simulink model "Taller1_SCADA"  (R2024a)
settings: Solver=VariableStepAuto  StartTime=0.0  StopTime=inf  RelTol=1e-3
libraries: spsThreePhaseTransformerTwoWindingsLib x2, spsThreePhaseVIMeasurementLib x2, spsPower3phInstantaneousLib x2, spsAsynchronousMachinepuUnitsLib x1, spsThreePhaseParallelRLCLoadLib x1, spsThreePhaseSeriesRLCBranchLib x1, spsThreePhaseBreakerLib x1, spsThreePhaseSourceLib x1, spsRMSLib x1, spspowerguiLib x1
settings Model: Creator=estudiante  LastModifiedBy=danan
settings SolverCC: AlgebraicLoopSolver=TrustRegion
settings DataIOCC: ReturnWorkspaceOutputs=off
settings DebuggingCC: UnconnectedInputMsg=warning  UnconnectedOutputMsg=warning  UnconnectedLineMsg=warning  ArithmeticOperatorsInVariantConditions=warning
settings ModelReferenceCC: EnableRefExpFcnMdlSchedulingChecks=on
settings SFSimCC: SimUseLocalCustomCode=off  CustomCodeUndefinedFunction=UseInterfaceOnly
settings RTWCC: RTWUseLocalCustomCode=off  GPUComputeCapability=3.5
settings CodeAppCC: StateflowObjectComments=on
settings SimscapeCC: SimscapeNormalizeSystem=off

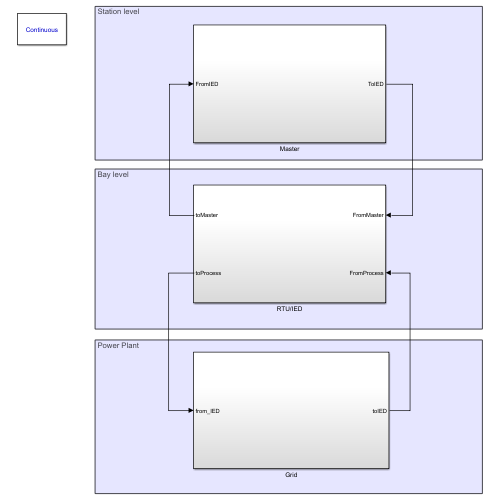
[thumbnail: Simulink's stored preview of the top-level diagram]
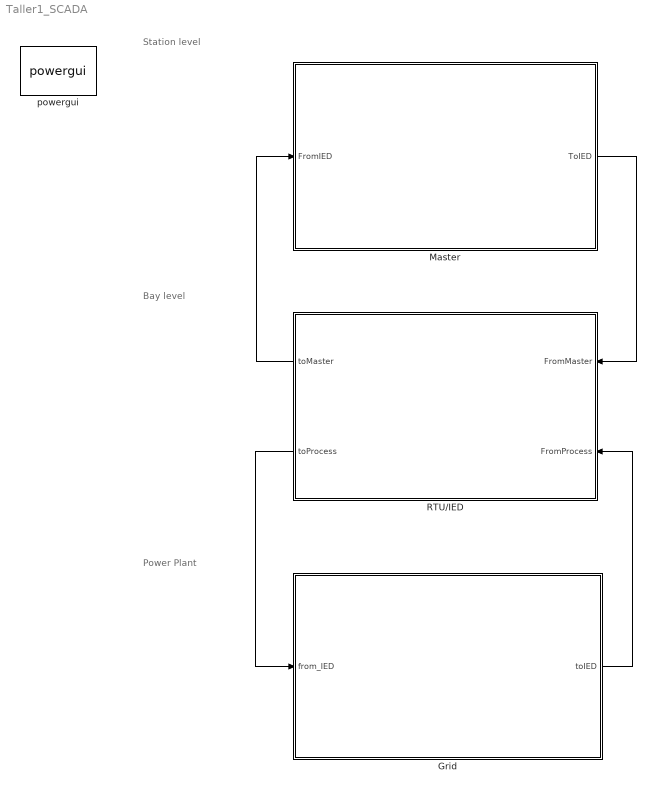
== system Taller1_SCADA ==
  note: Station level
  note: Bay level
  note: Power Plant
  Grid : Subsystem
  Master : Subsystem
  RTU/IED : Subsystem
  powergui : spspowerguiLib/powergui  Priority=1  SimulationMode=Continuous  SampleTime=50e-6  frequency=60  Iterations=50  frequencyindice=60  Pbase=100e6  ErrMax=1e-4  UnitsV=kV  UnitsW=MW  buscounter=0  FunctionMessages=off  echomessages=off  EnableUseOfTLC=off  CurrentSourceSwitches=off  DisableSnubberDevices=off  DisableRonSwitches=off  DisableVfSwitches=off  DisplayEquations=off  AutomaticDiscreteSolvers=off  SolverType=Tustin/Backward Euler (TBE)  Interpol=off  ExternalGateDelay=off  methode=off  Ts=10  x0status=blocks  SPID=off  SwTol=0  HookPort=off  NonlinearTolerance=1e-4  nMaxIteration=100  ContinueOnMaxIteration=off  RestoreLinks=warning  ResistiveCurrentMeasurement=off  Frange=[0:2:500]  Ylog=off  Xlog=on  ShowGrid=off  save=off  variable=ZData  structure=0  ZoomFFT=off  StartTime=0.0  cycles=1  DisplayStyle=1  fundamental=60  FreqAxis=off  MaxFrequency=1000  frequencyindicesteady=1  RmsSteady=1  display=off
  wires:
  RTU/IED/2(toProcess) -> Grid/1(from_IED)
  Grid/1(toIED) -> RTU/IED/2(FromProcess)
  RTU/IED/1(toMaster) -> Master/1(FromIED)
  Master/1(ToIED) -> RTU/IED/1(FromMaster)

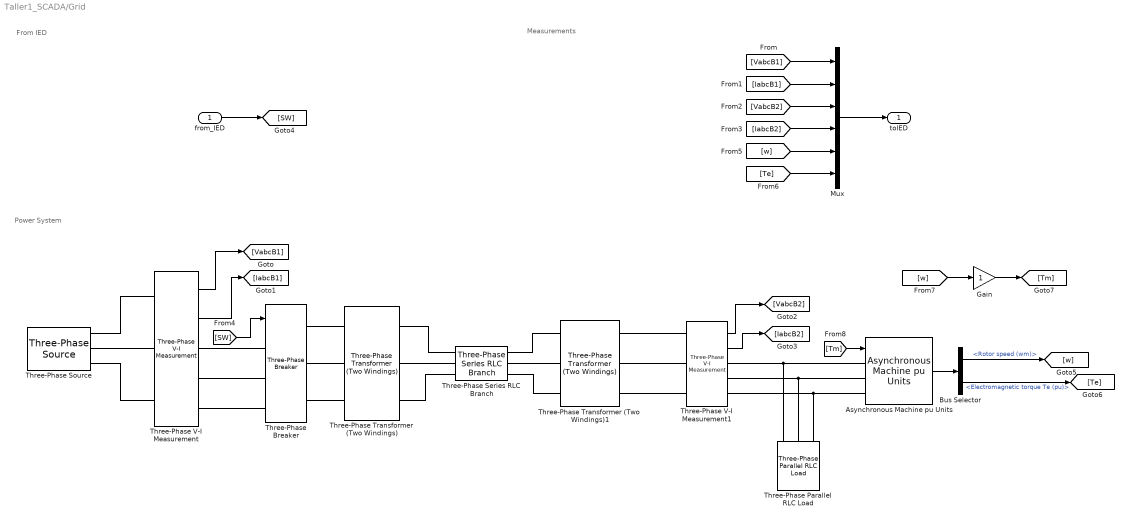
== system Taller1_SCADA/Grid ==
  note: From IED
  note: Measurements
  note: Power System
  from_IED : Inport
  Asynchronous Machine pu Units : spsAsynchronousMachinepuUnitsLib/Asynchronous Machine pu Units  RotorType=Squirrel-cage  PresetModel=No  MechanicalLoad=Torque Tm  ShowDetailedParameters=on  ReferenceFrame=Rotor  Units=pu  MeasurementBus=off  NominalParameters=[3730 460 60]  VoltageRatio=1  Stator=[0.01965 0.0397]  Rotor=[0.01909 0.0397]  Cage1=[0.01909 0.0397]  Cage2=[0.01909 0.0397]  Lm=1.354  Mechanical=[0.09526 0.05479 2]  PolePairs=2  InitialConditions="[ 1,0   0,0,0   0,0,0 ]"  SimulateSaturation=off  Saturation="[0.212,0.4201,0.8125,1.0979,1.4799,2.2457,3.2586,4.5763,6.4763 ;   0.5,0.7,0.9,1,1.1,1.2 ,1.3,1.4,1.5]"  LoadFlowParameters=0  TsPowergui=0  TsBlock=-1  IterativeModel=Trapezoidal non iterative  IterativeDiscreteModel=Trapezoidal non iterative  Pmec=0
      settings: LibrarySourceBlock=|
      | sps_lib/Electrical Machines/Asynchronous Machine
      | pu Units
  Bus Selector : BusSelector  OutputSignals=Mechanical.Rotor speed (wm),Mechanical.Electromagnetic torque Te (pu)
  Gain : Gain
  Mux : Mux  Inputs=6
  Three-Phase Parallel RLC Load : spsThreePhaseParallelRLCLoadLib/Three-Phase Parallel RLC Load  LConnTagsString=A|B|C  Configuration=Y (grounded)  NominalVoltage=1000  Vabc=[1e3 1e3 1e3]  Vabcp=[1e3 1e3 1e3]  NominalFrequency=60  UnbalancedPower=off  ActivePower=10e3  InductivePower=100  CapacitivePower=100  Pabc=[10e3 9e3 11e3]  QLabc=[100 90 110]  QCabc=[100 90 110]  Pabcp=[10e3 9e3 11e3]  QLabcp=[100 90 110]  QCabcp=[100 90 110]  Measurements=None  LoadType=constant Z
  Three-Phase Series RLC Branch : spsThreePhaseSeriesRLCBranchLib/Three-Phase Series RLC Branch  LConnTagsString=A|B|C  RConnTagsString=A|B|C  BranchType=RLC  Resistance=1  Inductance=1e-3  Capacitance=1e-6  Measurements=None
  Three-Phase Transformer (Two Windings) : spsThreePhaseTransformerTwoWindingsLib/Three-Phase Transformer (Two Windings)  Winding1Connection=Yg  Winding2Connection=Yg  CoreType=Three single-phase transformers  SetSaturation=off  Hysteresis=off  DataFile='hysteresis'  SetInitialFlux=off  Measurements=None  UNITS=pu  NominalPower=[ 250e6 , 60 ]  Winding1=[ 735e3 , 0.002 , 0.08 ]  Winding2=[ 315e3 , 0.002 , 0.08 ]  Rm=500  Lm=500  L0=0.5  Saturation=[ 0,0 ; 0.0024,1.2 ; 1.0,1.52 ]  InitialFluxes=[ 0.8 , -0.8 , 0.7 ]  BreakLoop=off  DiscreteSolver=Trapezoidal iterative  DataType=off  TransfoNumber=1
  Three-Phase Transformer (Two Windings)1 : spsThreePhaseTransformerTwoWindingsLib/Three-Phase Transformer (Two Windings)  Winding1Connection=Yg  Winding2Connection=Yg  CoreType=Three single-phase transformers  SetSaturation=off  Hysteresis=off  DataFile='hysteresis'  SetInitialFlux=off  Measurements=None  UNITS=pu  NominalPower=[ 250e6 , 60 ]  Winding1=[ 735e3 , 0.002 , 0.08 ]  Winding2=[ 315e3 , 0.002 , 0.08 ]  Rm=500  Lm=500  L0=0.5  Saturation=[ 0,0 ; 0.0024,1.2 ; 1.0,1.52 ]  InitialFluxes=[ 0.8 , -0.8 , 0.7 ]  BreakLoop=off  DiscreteSolver=Trapezoidal iterative  DataType=off  TransfoNumber=1
  Three-Phase V-I Measurement : spsThreePhaseVIMeasurementLib/Three-Phase V-I Measurement  VoltageMeasurement=phase-to-ground  SetLabelV=off  LabelV=Vabc  Vpu=off  VpuLL=off  CurrentMeasurement=yes  SetLabelI=off  LabelI=Iabc  Ipu=off  Pbase=100e6  Vbase=500e3  OutputType=Complex  PhasorSimulation=off  PSBequivalent=0
  Three-Phase V-I Measurement1 : spsThreePhaseVIMeasurementLib/Three-Phase V-I Measurement  VoltageMeasurement=phase-to-ground  SetLabelV=off  LabelV=Vabc  Vpu=off  VpuLL=off  CurrentMeasurement=yes  SetLabelI=off  LabelI=Iabc  Ipu=off  Pbase=100e6  Vbase=500e3  OutputType=Complex  PhasorSimulation=off  PSBequivalent=0
  Three-Phase Breaker : spsThreePhaseBreakerLib/Three-Phase Breaker  InitialState=open  SwitchA=on  SwitchB=on  SwitchC=on  SwitchTimes="[1/60  5/60]"  External=on  BreakerResistance=0.01  SnubberResistance=1e6  SnubberCapacitance=inf  Measurements=None
  Three-Phase Source : spsThreePhaseSourceLib/Three-Phase Source  InternalConnection=Yg  VoltagePhases=off  Voltage=25e3  PhaseAngle=0  Voltage_phases=[25e3 25e3 25e3]/sqrt(3)  PhaseAngles_phases=[0 -120 +120]  Frequency=60  NonIdealSource=on  SpecifyImpedance=off  Resistance=0.8929  Inductance=16.58e-3  ShortCircuitLevel=100e6  BaseVoltage=25e3  XRratio=7  BusType=swing  Pref=10e3  Qref=0  Prefabc=[10e3, 10e3, 10e3]  Qrefabc=[0, 0, 0]  Qmin=-inf  Qmax=inf
  toIED : Outport
  wires:
  Three-Phase V-I Measurement/1 -> [VabcB1]
  Three-Phase V-I Measurement/2 -> [IabcB1]
  Three-Phase V-I Measurement1/2 -> [IabcB2]
  Three-Phase V-I Measurement1/1 -> [VabcB2]
  Asynchronous Machine pu Units/1 -> Bus Selector/1
  [SW] -> Three-Phase Breaker/1
  Bus Selector/1 -> [w]  "<Rotor speed (wm)>"
  Bus Selector/2 -> [Te]  "<Electromagnetic torque Te (pu)>"
  from_IED/1 -> [SW]
  Mux/1 -> toIED/1
  [VabcB1] -> Mux/1
  [IabcB1] -> Mux/2
  [VabcB2] -> Mux/3
  [IabcB2] -> Mux/4
  [w] -> Mux/5
  [Te] -> Mux/6
  [w] -> Gain/1
  Gain/1 -> [Tm]
  [Tm] -> Asynchronous Machine pu Units/1
  connections:
  Three-Phase V-I Measurement/RConn3 -- Three-Phase Breaker/LConn3
  Three-Phase Transformer (Two Windings)/LConn1 -- Three-Phase Breaker/RConn1
  Three-Phase Source/RConn2 -- Three-Phase V-I Measurement/LConn2
  Three-Phase Breaker/RConn3 -- Three-Phase Transformer (Two Windings)/LConn3
  Three-Phase Transformer (Two Windings)/LConn2 -- Three-Phase Breaker/RConn2
  Three-Phase Transformer (Two Windings)1/LConn2 -- Three-Phase Series RLC Branch/RConn2
  Three-Phase Series RLC Branch/LConn1 -- Three-Phase Transformer (Two Windings)/RConn1
  Three-Phase Source/RConn1 -- Three-Phase V-I Measurement/LConn1
  Three-Phase Series RLC Branch/RConn1 -- Three-Phase Transformer (Two Windings)1/LConn1
  Three-Phase Source/RConn3 -- Three-Phase V-I Measurement/LConn3
  Three-Phase V-I Measurement/RConn1 -- Three-Phase Breaker/LConn1
  Three-Phase V-I Measurement/RConn2 -- Three-Phase Breaker/LConn2
  Three-Phase Series RLC Branch/LConn2 -- Three-Phase Transformer (Two Windings)/RConn2
  Three-Phase Series RLC Branch/LConn3 -- Three-Phase Transformer (Two Windings)/RConn3
  Three-Phase Series RLC Branch/RConn3 -- Three-Phase Transformer (Two Windings)1/LConn3
  Asynchronous Machine pu Units/LConn1 -- Three-Phase Parallel RLC Load/LConn1 -- Three-Phase V-I Measurement1/RConn1
  Asynchronous Machine pu Units/LConn2 -- Three-Phase Parallel RLC Load/LConn2 -- Three-Phase V-I Measurement1/RConn2
  Asynchronous Machine pu Units/LConn3 -- Three-Phase Parallel RLC Load/LConn3 -- Three-Phase V-I Measurement1/RConn3
  Three-Phase V-I Measurement1/LConn1 -- Three-Phase Transformer (Two Windings)1/RConn1
  Three-Phase V-I Measurement1/LConn2 -- Three-Phase Transformer (Two Windings)1/RConn2
  Three-Phase V-I Measurement1/LConn3 -- Three-Phase Transformer (Two Windings)1/RConn3

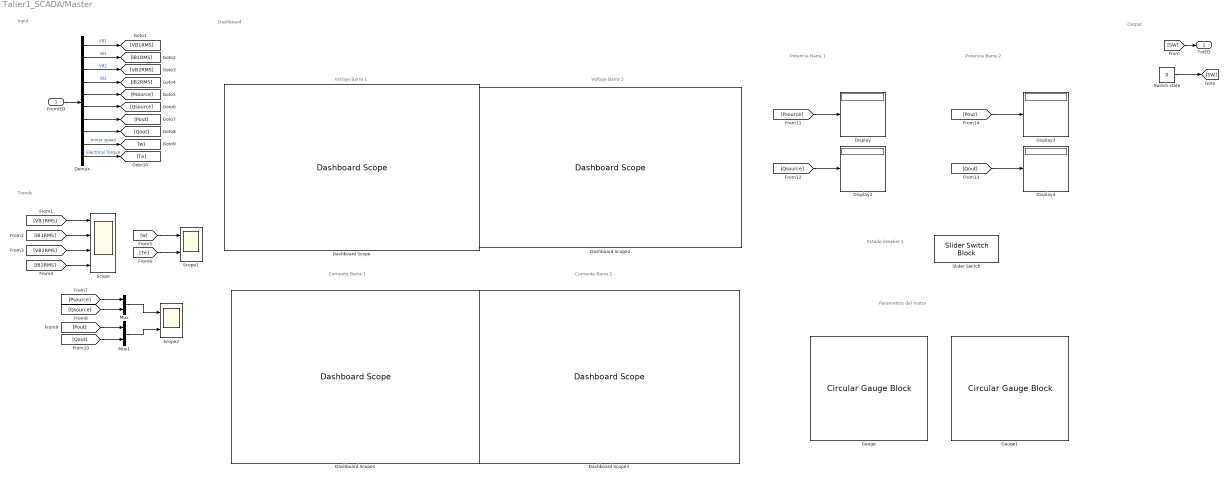
== system Taller1_SCADA/Master ==
  note: Voltaje Barra 1
  note: Dashboard
  note: Output
  note: Trends
  note: Input
  note: Voltaje Barra 2
  note: Corriente Barra 1
  note: Corriente Barra 2
  note: Potencia Barra 1
  note: Estado breaker 1
  note: Potencia Barra 2
  note: Parametros del motor
  FromIED : Inport
  Dashboard Scope{,1..3} (4 alike) : DashboardScope
  Demux : Demux  Outputs=10
  Display{,2..4} (4 alike) : Display
  Gauge : CircularGaugeBlock
  Gauge1 : CircularGaugeBlock
  Mux : Mux  Inputs=2
  Mux1 : Mux  Inputs=2
  Scope : Scope  NumInputPorts=4
  Scope1 : Scope  NumInputPorts=2
  Scope2 : Scope  NumInputPorts=2
  Slider Switch : SliderSwitchBlock
      settings: Values={{'Off', 'On'}, [0 1]}
  Switch state : Constant  Value=0
  ToIED : Outport
  wires:
  Switch state/1 -> [SW]
  [SW] -> ToIED/1
  FromIED/1 -> Demux/1
  Demux/1 -> [VB1RMS]  "VB1"
  Demux/2 -> [IB1RMS]  "IB1"
  Demux/4 -> [IB2RMS]  "IB2"
  Demux/3 -> [VB2RMS]  "VB2"
  Demux/8 -> [Qout]
  Demux/7 -> [Pout]
  Demux/6 -> [Qsource]
  Demux/5 -> [Psource]
  Demux/9 -> [w]  "motor speed"
  Demux/10 -> [Te]  "Electrical Torque"
  [IB2RMS] -> Scope/4
  [VB2RMS] -> Scope/3
  [IB1RMS] -> Scope/2
  [VB1RMS] -> Scope/1
  [Te] -> Scope1/2
  [w] -> Scope1/1
  [Psource] -> Mux/1
  [Qsource] -> Mux/2
  [Pout] -> Mux1/1
  [Qout] -> Mux1/2
  Mux/1 -> Scope2/1
  Mux1/1 -> Scope2/2
  [Psource] -> Display/1
  [Qsource] -> Display2/1
  [Pout] -> Display3/1
  [Qout] -> Display4/1

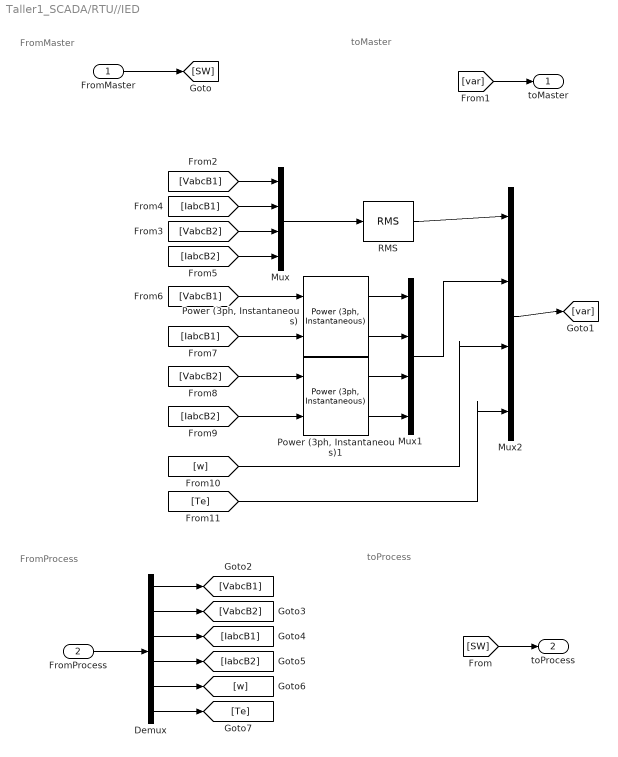
== system Taller1_SCADA/RTU//IED ==
  note: toProcess
  note: FromProcess
  note: toMaster
  note: FromMaster
  FromMaster : Inport
  FromProcess : Inport  Port=2
  Demux : Demux  Outputs=6
  Mux : Mux
  Mux1 : Mux
  Mux2 : Mux
  "Power (3ph, Instantaneous)" : spsPower3phInstantaneousLib/Power (3ph, Instantaneous)
  "Power (3ph, Instantaneous)1" : spsPower3phInstantaneousLib/Power (3ph, Instantaneous)
  RMS : spsRMSLib/RMS  TrueRMS=on  Freq=60  RMSInit=120  Ts=0
  toMaster : Outport
  toProcess : Outport  Port=2
  wires:
  FromMaster/1 -> [SW]
  [SW] -> toProcess/1
  Mux/1 -> RMS/1
  "Power (3ph, Instantaneous)"/1 -> Mux1/1
  "Power (3ph, Instantaneous)"/2 -> Mux1/2
  "Power (3ph, Instantaneous)1"/1 -> Mux1/3
  "Power (3ph, Instantaneous)1"/2 -> Mux1/4
  [var] -> toMaster/1
  Demux/1 -> [VabcB1]
  Demux/2 -> [VabcB2]
  Demux/3 -> [IabcB1]
  Demux/4 -> [IabcB2]
  Demux/5 -> [w]
  Demux/6 -> [Te]
  FromProcess/1 -> Demux/1
  [VabcB1] -> Mux/1
  [VabcB2] -> Mux/3
  [IabcB2] -> Mux/4
  [IabcB1] -> Mux/2
  [VabcB1] -> "Power (3ph, Instantaneous)"/1
  [IabcB1] -> "Power (3ph, Instantaneous)"/2
  [VabcB2] -> "Power (3ph, Instantaneous)1"/1
  [IabcB2] -> "Power (3ph, Instantaneous)1"/2
  RMS/1 -> Mux2/1
  Mux2/1 -> [var]
  Mux1/1 -> Mux2/2
  [w] -> Mux2/3
  [Te] -> Mux2/4
